simulink model "paramAB_model"  (Simulink 9.3)
settings: Solver=ode23s  StartTime=0.0  StopTime=8  RelTol=1e-3  EnableMultiTasking=on
values from neighbouring files (symbols this model uses):
  model = init_param.model    [paramAB_MPC.m]
undefined symbols (not defined in the file or in its folder): control, simulate
settings Model: Creator=johwa  LastModifiedBy=Jonte  ExtModeAutoUpdateStatusClock=off
settings SolverCC: ConsecutiveZCsStepRelTol=eps
settings DataIOCC: SaveFinalState=on  SignalLoggingName=sigsOut
settings OptimizationCC: ExpressionDepthLimit=2147483647  InitFltsAndDblsToZero=on
settings DebuggingCC: SaveWithParameterizedLinksMsg=none  SignalResolutionControl=TryResolveAllWithWarning  MultiTaskDSMMsg=warning  MultiTaskCondExecSysMsg=none  StateNameClashWarn=warning
settings HardwareCC: TargetUnknown=on
settings GRTTargetCC: TargetFcnLib=ansi_tfl_tmw.mat  GeneratePreprocessorConditionals=Disable all

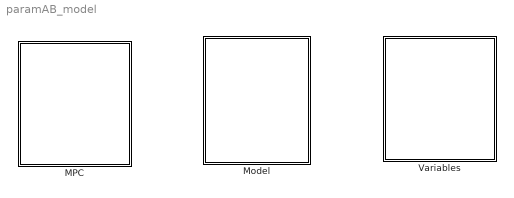
== system paramAB_model ==
  MPC : Subsystem
  Model : Subsystem
  Variables : Subsystem

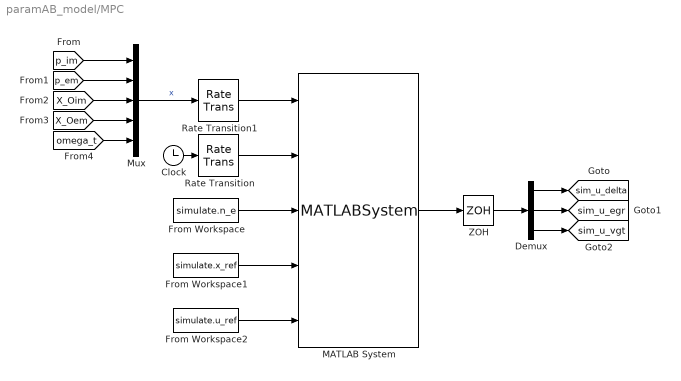
== system paramAB_model/MPC ==
  Clock : Clock
  Demux : Demux  Outputs=3
  From Workspace : FromWorkspace  VariableName=simulate.n_e  SampleTime=simulate.T_s  Interpolate=off  OutputAfterFinalValue=Holding final value
  From Workspace1 : FromWorkspace  VariableName=simulate.x_ref  SampleTime=simulate.T_s  Interpolate=off  OutputAfterFinalValue=Holding final value
  From Workspace2 : FromWorkspace  VariableName=simulate.u_ref  SampleTime=simulate.T_s  Interpolate=off  OutputAfterFinalValue=Holding final value
  MATLAB System : MATLABSystem  System=paramAB_MPC  SimulateUsing=Interpreted execution
      mask Type: paramAB_MPC
      mask Display:
      | disp('paramAB_MPC');
      | port_label('input',1,'x');
      | port_label('input',2,'t');
      | port_label('input',3,'n_e');
      | port_label('input',4,'x_ref');
      | port_label('input',5,'u_ref');
      | port_label('output',1,'u');
  Mux : Mux  Inputs=5
  Rate Transition : RateTransition  OutPortSampleTime=simulate.T_s
  Rate Transition1 : RateTransition  OutPortSampleTime=simulate.T_s
  ZOH : ZeroOrderHold  SampleTime=simulate.T_s
  tag scope: sim_u_delta=global, sim_u_egr=global, sim_u_vgt=global
  wires:
  [omega_t] -> Mux/5
  [X_Oim] -> Mux/3
  [p_im] -> Mux/1
  [p_em] -> Mux/2
  [X_Oem] -> Mux/4
  Clock/1 -> Rate Transition/1
  Rate Transition/1 -> MATLAB System/2
  Demux/2 -> [sim_u_egr]
  Demux/1 -> [sim_u_delta]
  Demux/3 -> [sim_u_vgt]
  MATLAB System/1 -> ZOH/1
  ZOH/1 -> Demux/1
  Mux/1 -> Rate Transition1/1  "x"
  Rate Transition1/1 -> MATLAB System/1
  From Workspace1/1 -> MATLAB System/4
  From Workspace2/1 -> MATLAB System/5
  From Workspace/1 -> MATLAB System/3

== system paramAB_model/Model ==
  Engine : Subsystem  mask{gamma_e=model.gamma_e, gamma_a=model.gamma_a, p_amb=model.p_amb, c_ve=model.c_ve, c_va=model.c_va, c_pe=model.c_pe, c_pa=model.c_pa, T_im=model.T_im, T_amb=model.T_amb, R_e=model.R_e, R_a=model.R_a, X_Oc=model.X_Oc}
      mask help:
      | A model for a Diesel engine with EGT and VGT.
      |
      | The model is develped and parameterized for a Scania heavy duty truck engine and documented in the paper:
      |
      | Johan Wahlstrom and Lars Eriksson.
      | Modeling diesel engines with a variable-geometry turbocharger and exhaust gas recirculation by optimization of model parameters for capturing non-linear system dynamics.
      | Proceedings of the Institution of Mechanical Engineers, Part D, Journal of Automobile Engineering, Volume 225, Issue 7, July 2011.
      | http://dx.doi.org/10.1177/0954407011398177
      mask Help: To see the details of the model right click on the model select "Look Under Mask".
  From Workspace3 : FromWorkspace  VariableName=simulate.n_e  SampleTime=0  Interpolate=off  OutputAfterFinalValue=Holding final value
  wires:
  From Workspace3/1 -> Engine/4(n_e)
  [sim_u_delta] -> Engine/3(u_delta)
  [sim_u_egr] -> Engine/2(u_egr)
  [sim_u_vgt] -> Engine/1(u_vgt)

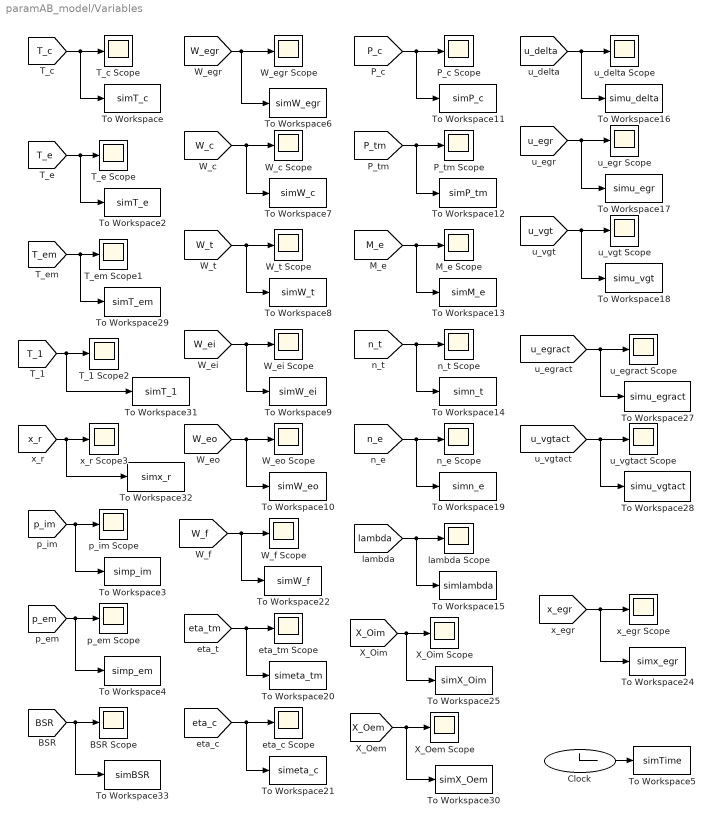
== system paramAB_model/Variables ==
  BSR Scope : Scope
  Clock : Clock
  M_e Scope : Scope
  P_c Scope : Scope
  P_tm Scope : Scope
  T_1 Scope2 : Scope
  T_c Scope : Scope
  T_e Scope : Scope
  T_em Scope1 : Scope
  To Workspace : ToWorkspace  VariableName=simT_c  SampleTime=-1
  To Workspace10 : ToWorkspace  VariableName=simW_eo  SampleTime=-1
  To Workspace11 : ToWorkspace  VariableName=simP_c  SampleTime=-1
  To Workspace12 : ToWorkspace  VariableName=simP_tm  SampleTime=-1
  To Workspace13 : ToWorkspace  VariableName=simM_e  SampleTime=-1
  To Workspace14 : ToWorkspace  VariableName=simn_t  SampleTime=-1
  To Workspace15 : ToWorkspace  VariableName=simlambda  SampleTime=-1
  To Workspace16 : ToWorkspace  VariableName=simu_delta  SampleTime=-1
  To Workspace17 : ToWorkspace  VariableName=simu_egr  SampleTime=-1
  To Workspace18 : ToWorkspace  VariableName=simu_vgt  SampleTime=-1
  To Workspace19 : ToWorkspace  VariableName=simn_e  SampleTime=-1
  To Workspace2 : ToWorkspace  VariableName=simT_e  SampleTime=-1
  To Workspace20 : ToWorkspace  VariableName=simeta_tm  SampleTime=-1
  To Workspace21 : ToWorkspace  VariableName=simeta_c  SampleTime=-1
  To Workspace22 : ToWorkspace  VariableName=simW_f  SampleTime=-1
  To Workspace24 : ToWorkspace  VariableName=simx_egr  SampleTime=-1
  To Workspace25 : ToWorkspace  VariableName=simX_Oim  SampleTime=-1
  To Workspace27 : ToWorkspace  VariableName=simu_egract  SampleTime=-1
  To Workspace28 : ToWorkspace  VariableName=simu_vgtact  SampleTime=-1
  To Workspace29 : ToWorkspace  VariableName=simT_em  SampleTime=-1
  To Workspace3 : ToWorkspace  VariableName=simp_im  SampleTime=-1
  To Workspace30 : ToWorkspace  VariableName=simX_Oem  SampleTime=-1
  To Workspace31 : ToWorkspace  VariableName=simT_1  SampleTime=-1
  To Workspace32 : ToWorkspace  VariableName=simx_r  SampleTime=-1
  To Workspace33 : ToWorkspace  VariableName=simBSR  SampleTime=-1
  To Workspace4 : ToWorkspace  VariableName=simp_em  SampleTime=-1
  To Workspace5 : ToWorkspace  VariableName=simTime  SampleTime=-1
  To Workspace6 : ToWorkspace  VariableName=simW_egr  SampleTime=-1
  To Workspace7 : ToWorkspace  VariableName=simW_c  SampleTime=-1
  To Workspace8 : ToWorkspace  VariableName=simW_t  SampleTime=-1
  To Workspace9 : ToWorkspace  VariableName=simW_ei  SampleTime=-1
  W_c Scope : Scope
  W_egr Scope : Scope
  W_ei Scope : Scope
  W_eo Scope : Scope
  W_f Scope : Scope
  W_t Scope : Scope
  X_Oem Scope : Scope
  X_Oim Scope : Scope
  eta_c Scope : Scope
  eta_tm Scope : Scope
  lambda Scope : Scope
  n_e Scope : Scope
  n_t Scope : Scope
  p_em Scope : Scope
  p_im Scope : Scope
  u_delta Scope : Scope
  u_egr Scope : Scope
  u_egract Scope : Scope
  u_vgt Scope : Scope
  u_vgtact Scope : Scope
  x_egr Scope : Scope
  x_r Scope3 : Scope
  wires:
  [u_vgtact] -> To Workspace28/1, u_vgtact Scope/1
  [u_egract] -> u_egract Scope/1, To Workspace27/1
  [x_egr] -> x_egr Scope/1, To Workspace24/1
  [W_f] -> W_f Scope/1, To Workspace22/1
  [eta_c] -> To Workspace21/1, eta_c Scope/1
  [eta_tm] -> eta_tm Scope/1, To Workspace20/1
  [n_e] -> n_e Scope/1, To Workspace19/1
  [u_vgt] -> u_vgt Scope/1, To Workspace18/1
  [u_egr] -> To Workspace17/1, u_egr Scope/1
  [u_delta] -> u_delta Scope/1, To Workspace16/1
  Clock/1 -> To Workspace5/1
  [lambda] -> To Workspace15/1, lambda Scope/1
  [M_e] -> To Workspace13/1, M_e Scope/1
  [W_eo] -> To Workspace10/1, W_eo Scope/1
  [P_tm] -> To Workspace12/1, P_tm Scope/1
  [P_c] -> To Workspace11/1, P_c Scope/1
  [W_ei] -> To Workspace9/1, W_ei Scope/1
  [W_t] -> To Workspace8/1, W_t Scope/1
  [W_c] -> To Workspace7/1, W_c Scope/1
  [W_egr] -> To Workspace6/1, W_egr Scope/1
  [n_t] -> To Workspace14/1, n_t Scope/1
  [p_em] -> To Workspace4/1, p_em Scope/1
  [p_im] -> To Workspace3/1, p_im Scope/1
  [T_e] -> To Workspace2/1, T_e Scope/1
  [T_c] -> To Workspace/1, T_c Scope/1
  [T_em] -> T_em Scope1/1, To Workspace29/1
  [X_Oem] -> X_Oem Scope/1, To Workspace30/1
  [X_Oim] -> X_Oim Scope/1, To Workspace25/1
  [T_1] -> T_1 Scope2/1, To Workspace31/1
  [x_r] -> x_r Scope3/1, To Workspace32/1
  [BSR] -> BSR Scope/1, To Workspace33/1

== system paramAB_model/Model/Engine ==
  u_vgt : Inport
  u_egr : Inport  Port=2
  u_delta : Inport  Port=3
  n_e : Inport  Port=4
  Cylinder : Subsystem  mask{n_cyl=model.n_cyl, AFs=model.AFs, q_HV=model.q_HV, V_d=model.V_d, r_c=model.r_c}
  EGR-system : Subsystem  mask{PI_egropt=model.PI_egropt, c_egr=model.c_egr, uInit_egr=simulate.u_egr_Init, A_egrmax=model.A_egrmax}
  Exhaust Manifold : Subsystem  mask{p_em_Init=simulate.p_em_Init, V_em=model.V_em}
  Inlet Manifold temp : Constant  Value=T_im
  Intake Manifold : Subsystem  mask{p_im_Init=simulate.p_im_Init, V_im=model.V_im}
  Turbo : Subsystem
  tag scope: T_c=global
  wires:
  Exhaust Manifold/2(X_Oem) -> Intake Manifold/5(X_Oem)
  Cylinder/4(X_Oe) -> Exhaust Manifold/5(X_Oe)
  Intake Manifold/2(X_Oim) -> Cylinder/3(X_Oim)
  u_delta/1 -> Cylinder/5(u_delta)
  n_e/1 -> Cylinder/4(n_e)
  Turbo/2(T_c) -> [T_c]
  u_vgt/1 -> Turbo/4(u_vgt)
  u_egr/1 -> EGR-system/4(u_egr)
  Cylinder/3(T_em) -> EGR-system/2(T_em), Turbo/3(T_em), Exhaust Manifold/4(T_em)
  Cylinder/1(W_ei) -> Intake Manifold/3(W_ei)
  Inlet Manifold temp/1 -> Intake Manifold/4(T_im), Cylinder/6(T_im)
  Turbo/1(W_c) -> Intake Manifold/1(W_c)
  EGR-system/1(W_egr) -> Intake Manifold/2(W_egr), Exhaust Manifold/3(W_egr)
  Turbo/3(W_t) -> Exhaust Manifold/2(W_t)
  Cylinder/2(W_eo) -> Exhaust Manifold/1(W_eo)
  Exhaust Manifold/1(p_em) -> EGR-system/3(p_em), Turbo/2(p_em), Cylinder/2(p_em)
  Intake Manifold/1(p_im) -> EGR-system/1(p_im), Turbo/1(p_im), Cylinder/1(p_im)

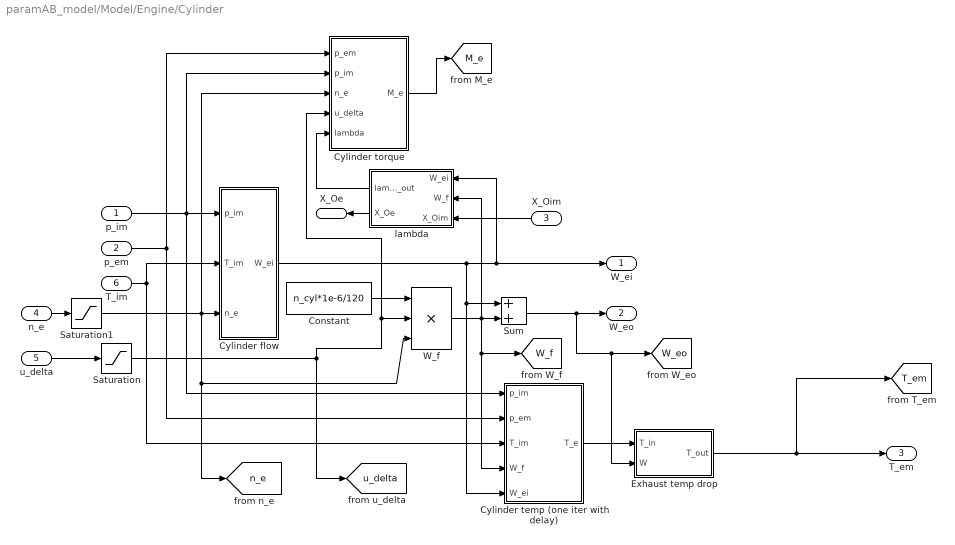
== system paramAB_model/Model/Engine/Cylinder ==
  p_im : Inport
  p_em : Inport  Port=2
  X_Oim : Inport  Port=3
  n_e : Inport  Port=4
  u_delta : Inport  Port=5
  T_im : Inport  Port=6
  Constant : Constant  Value=n_cyl*1e-6/120
  Cylinder flow : Subsystem  mask{c_volVec=model.c_volVec}
  Cylinder temp (one iter with delay) : Subsystem  mask{x_cv=model.x_cv, eta_sc=model.eta_sc, x_r_Init=simulate.x_r_Init, T_1_Init=simulate.T_1_Init}
  Cylinder torque : Subsystem  mask{c_fricVec=model.c_fricVec, eta_igch=model.eta_igch, gamma_c=model.gamma_c}
  Exhaust temp drop : Subsystem  mask{h_tot=model.h_tot, n_pipe=model.n_pipe, l_pipe=model.l_pipe, d_pipe=model.d_pipe, T_w=model.T_w}
  Saturation : Saturate  UpperLimit=250  LowerLimit=1
  Saturation1 : Saturate  UpperLimit=2000  LowerLimit=500
  Sum : Sum  SaturateOnIntegerOverflow=on
  W_f : Product  Inputs=3  SaturateOnIntegerOverflow=on  OutDataTypeStr=Inherit: Same as first input
  lambda : Subsystem
  W_ei : Outport
  W_eo : Outport  Port=2
  T_em : Outport  Port=3
  X_Oe : Outport  Port=4
  tag scope: M_e=global, T_em=global, W_eo=global, W_f=global, n_e=global, u_delta=global
  wires:
  Saturation/1 -> W_f/2, Cylinder torque/4(u_delta), [u_delta]
  lambda/2(X_Oe) -> X_Oe/1
  n_e/1 -> Saturation1/1
  X_Oim/1 -> lambda/3(X_Oim)
  lambda/1(lambda_out) -> Cylinder torque/5(lambda)
  Cylinder temp (one iter with delay)/1(T_e) -> Exhaust temp drop/1(T_in)
  Cylinder torque/1(M_e) -> [M_e]
  u_delta/1 -> Saturation/1
  Constant/1 -> W_f/1
  W_f/1 -> lambda/2(W_f), [W_f], Cylinder temp (one iter with delay)/4(W_f), Sum/2
  Sum/1 -> Exhaust temp drop/2(W), [W_eo], W_eo/1
  Cylinder flow/1(W_ei) -> lambda/1(W_ei), W_ei/1, Cylinder temp (one iter with delay)/5(W_ei), Sum/1
  T_im/1 -> Cylinder flow/2(T_im), Cylinder temp (one iter with delay)/3(T_im)
  p_em/1 -> Cylinder torque/1(p_em), Cylinder temp (one iter with delay)/2(p_em)
  p_im/1 -> Cylinder torque/2(p_im), Cylinder temp (one iter with delay)/1(p_im), Cylinder flow/1(p_im)
  Exhaust temp drop/1(T_out) -> [T_em], T_em/1
  Saturation1/1 -> Cylinder flow/3(n_e), [n_e], W_f/3, Cylinder torque/3(n_e)

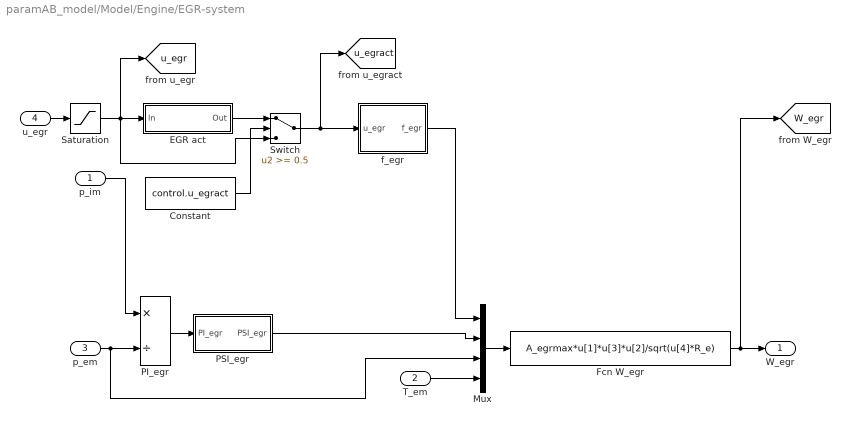
== system paramAB_model/Model/Engine/EGR-system ==
  p_im : Inport
  T_em : Inport  Port=2
  p_em : Inport  Port=3
  u_egr : Inport  Port=4
  Constant : Constant  Value=control.u_egract
  EGR act : Subsystem
  Fcn W_egr : Fcn  Expr=A_egrmax*u[1]*u[3]*u[2]/sqrt(u[4]*R_e)
  Mux : Mux
  PI_egr : Product  Inputs=*/  SaturateOnIntegerOverflow=on  OutDataTypeStr=Inherit: Same as first input
  PSI_egr : Subsystem
  Saturation : Saturate  UpperLimit=100  LowerLimit=0
  Switch : Switch  Threshold=0.5  SaturateOnIntegerOverflow=on
  f_egr : Subsystem
  W_egr : Outport
  tag scope: W_egr=global, u_egr=global, u_egract=global
  wires:
  Constant/1 -> Switch/2
  EGR act/1(Out) -> Switch/1
  Switch/1 -> [u_egract], f_egr/1(u_egr)
  u_egr/1 -> Saturation/1
  Fcn W_egr/1 -> [W_egr], W_egr/1
  T_em/1 -> Mux/4
  PSI_egr/1(PSI_egr) -> Mux/2
  f_egr/1(f_egr) -> Mux/1
  Mux/1 -> Fcn W_egr/1
  PI_egr/1 -> PSI_egr/1(PI_egr)
  p_em/1 -> Mux/3, PI_egr/2
  p_im/1 -> PI_egr/1
  Saturation/1 -> EGR act/1(In), Switch/3, [u_egr]

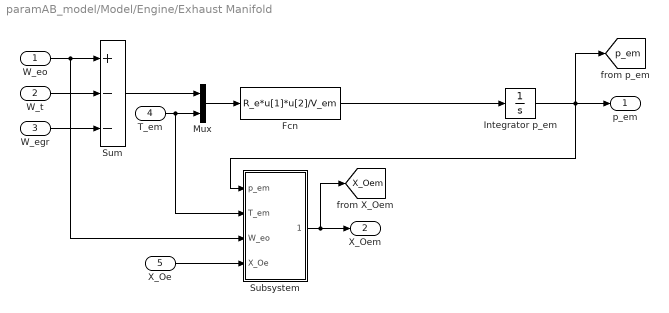
== system paramAB_model/Model/Engine/Exhaust Manifold ==
  W_eo : Inport
  W_t : Inport  Port=2
  W_egr : Inport  Port=3
  T_em : Inport  Port=4
  X_Oe : Inport  Port=5
  Fcn : Fcn  Expr=R_e*u[1]*u[2]/V_em
  Integrator p_em : Integrator  InitialCondition=p_em_Init  LimitOutput=on  UpperSaturationLimit=20*p_amb  LowerSaturationLimit=0.5*p_amb
  Mux : Mux  Inputs=2
  Subsystem : Subsystem
  Sum : Sum  Inputs=+--  SaturateOnIntegerOverflow=on
  p_em : Outport
  X_Oem : Outport  Port=2
  tag scope: X_Oem=global, p_em=global
  wires:
  Subsystem/1(X_Oem) -> [X_Oem], X_Oem/1
  X_Oe/1 -> Subsystem/4(X_Oe)
  Integrator p_em/1 -> Subsystem/1(p_em), [p_em], p_em/1
  W_eo/1 -> Subsystem/3(W_eo), Sum/1
  W_t/1 -> Sum/2
  W_egr/1 -> Sum/3
  Sum/1 -> Mux/1
  T_em/1 -> Subsystem/2(T_em), Mux/2
  Mux/1 -> Fcn/1
  Fcn/1 -> Integrator p_em/1

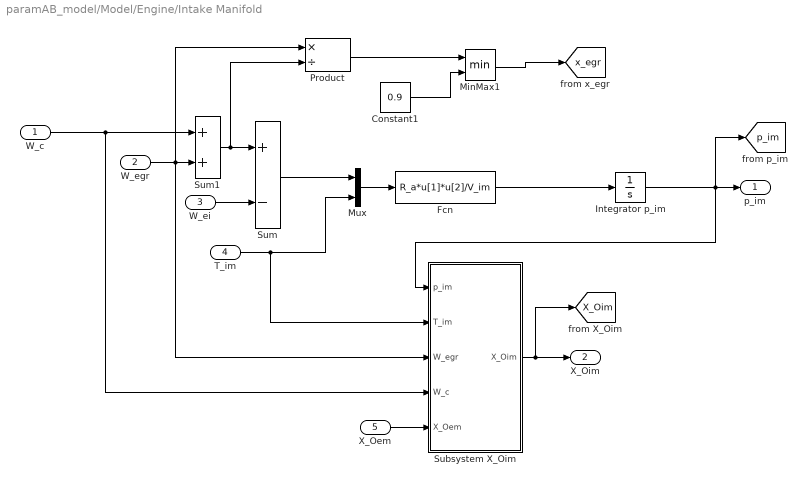
== system paramAB_model/Model/Engine/Intake Manifold ==
  W_c : Inport
  W_egr : Inport  Port=2
  W_ei : Inport  Port=3
  T_im : Inport  Port=4
  X_Oem : Inport  Port=5
  Constant1 : Constant  Value=0.9
  Fcn : Fcn  Expr=R_a*u[1]*u[2]/V_im
  Integrator p_im : Integrator  InitialCondition=p_im_Init  LimitOutput=on  UpperSaturationLimit=10*p_amb  LowerSaturationLimit=0.5*p_amb
  MinMax1 : MinMax  Inputs=2  SaturateOnIntegerOverflow=on  InputSameDT=on
  Mux : Mux  Inputs=2
  Product : Product  Inputs=*/  SaturateOnIntegerOverflow=on  OutDataTypeStr=Inherit: Same as first input
  Subsystem X_Oim : Subsystem
  Sum : Sum  Inputs=+-  SaturateOnIntegerOverflow=on
  Sum1 : Sum  SaturateOnIntegerOverflow=on
  p_im : Outport
  X_Oim : Outport  Port=2
  tag scope: X_Oim=global, p_im=global, x_egr=global
  wires:
  Subsystem X_Oim/1(X_Oim) -> [X_Oim], X_Oim/1
  X_Oem/1 -> Subsystem X_Oim/5(X_Oem)
  Product/1 -> MinMax1/1
  Constant1/1 -> MinMax1/2
  W_egr/1 -> Subsystem X_Oim/3(W_egr), Product/1, Sum1/2
  W_c/1 -> Subsystem X_Oim/4(W_c), Sum1/1
  Sum1/1 -> Product/2, Sum/1
  Fcn/1 -> Integrator p_im/1
  Mux/1 -> Fcn/1
  T_im/1 -> Subsystem X_Oim/2(T_im), Mux/2
  Sum/1 -> Mux/1
  W_ei/1 -> Sum/2
  Integrator p_im/1 -> Subsystem X_Oim/1(p_im), [p_im], p_im/1
  MinMax1/1 -> [x_egr]

== system paramAB_model/Model/Engine/Turbo ==
  p_im : Inport
  p_em : Inport  Port=2
  T_em : Inport  Port=3
  u_vgt : Inport  Port=4
  Compressor : Subsystem  mask{c_pi=model.c_pi, pi_copt=model.pi_copt, w_copt=model.w_copt, eta_cmax=model.eta_cmax, Q_c=model.Q_c, c_wphiVec=model.c_wphiVec, c_wpsiVec=model.c_wpsiVec, c_phi2=model.c_phi2, c_psi2=model.c_psi2, R_c=model.R_c}
  Turbine : Subsystem  mask{c_vgt2=model.c_vgt2, c_vgt1=model.c_vgt1, c_f2=model.c_f2, c_f1=model.c_f1, K_t=model.K_t, uInit_vgt=simulate.u_vgt_Init, tau_vgt=model.tau_vgt, c_mlin=model.c_mlin, w_tlin=model.w_tlin, c_mVec=model.c_mVec, BSR_opt=model.BSR_opt, eta_tmmax=model.eta_tmmax, R_t=model.R_t, A_vgtmax=model.A_vgtmax}
  Turbo inertia : Subsystem  mask{omega_t_Init=simulate.omega_t_Init, J_t=model.J_t}
  amb pres : Constant  Value=p_amb
  amb temp : Constant  Value=T_amb
  W_c : Outport
  T_c : Outport  Port=2
  W_t : Outport  Port=3
  wires:
  u_vgt/1 -> Turbine/5(u_vgt)
  T_em/1 -> Turbine/1(T_em)
  p_em/1 -> Turbine/2(p_em)
  Turbine/1(W_t) -> W_t/1
  Compressor/2(T_c) -> T_c/1
  Compressor/1(W_c) -> W_c/1
  Compressor/3(P_c) -> Turbo inertia/2(P_c)
  Turbine/2(P_t*eta_m) -> Turbo inertia/1(P_t*eta_m)
  Turbo inertia/1(omega_t) -> Turbine/4(omega_t), Compressor/4(omega_t)
  p_im/1 -> Compressor/3(p_c)
  amb pres/1 -> Turbine/3(p_es), Compressor/2(p_bc)
  amb temp/1 -> Compressor/1(T_bc)

== system paramAB_model/Model/Engine/Cylinder/Cylinder flow ==
  p_im : Inport
  T_im : Inport  Port=2
  n_e : Inport  Port=3
  Constant : Constant  Value=V_d/(R_a*60*2)
  Mux : Mux  Inputs=2
  Product W_ei : Product  Inputs=***/*  SaturateOnIntegerOverflow=on  OutDataTypeStr=Inherit: Same as first input
  n_vol : Fcn  Expr=c_volVec(1)*sqrt(u[1])+c_volVec(2)*sqrt(u[2])+c_volVec(3)
  W_ei : Outport
  tag scope: W_ei=global
  wires:
  Mux/1 -> n_vol/1
  Product W_ei/1 -> [W_ei], W_ei/1
  Constant/1 -> Product W_ei/5
  T_im/1 -> Product W_ei/4
  n_e/1 -> Mux/2, Product W_ei/3
  n_vol/1 -> Product W_ei/1
  p_im/1 -> Mux/1, Product W_ei/2

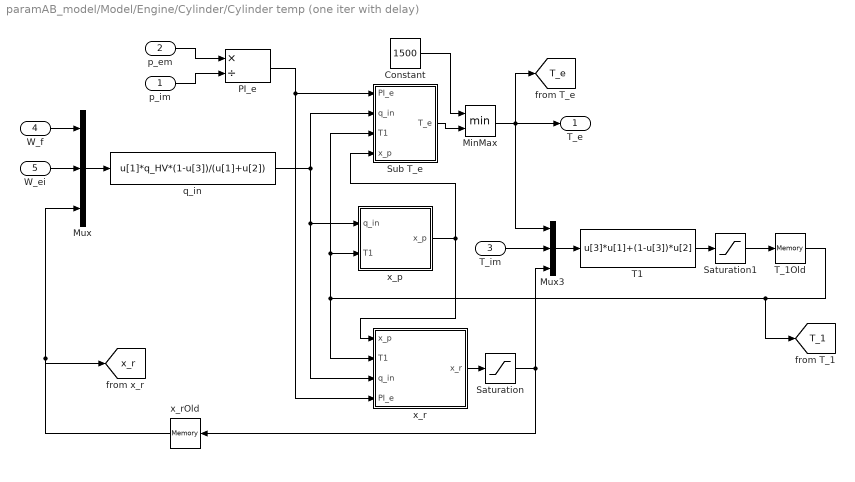
== system paramAB_model/Model/Engine/Cylinder/Cylinder temp (one iter with delay) ==
  p_im : Inport
  p_em : Inport  Port=2
  T_im : Inport  Port=3
  W_f : Inport  Port=4
  W_ei : Inport  Port=5
  Constant : Constant  Value=1500
  MinMax : MinMax  Inputs=2  SaturateOnIntegerOverflow=on  InputSameDT=on
  Mux : Mux  Inputs=3
  Mux3 : Mux  Inputs=3
  PI_e : Product  Inputs=*/  SaturateOnIntegerOverflow=on  OutDataTypeStr=Inherit: Same as first input
  Saturation : Saturate  UpperLimit=1  LowerLimit=0
  Saturation1 : Saturate  UpperLimit=inf  LowerLimit=273
  Sub T_e : Subsystem
  T1 : Fcn  Expr=u[3]*u[1]+(1-u[3])*u[2]
  T_1Old : Memory  InitialCondition=T_1_Init  InheritSampleTime=on
  q_in : Fcn  Expr=u[1]*q_HV*(1-u[3])/(u[1]+u[2])
  x_p : Subsystem
  x_r : Subsystem
  x_rOld : Memory  InitialCondition=x_r_Init  InheritSampleTime=on
  T_e : Outport
  tag scope: T_1=global, T_e=global, x_r=global
  wires:
  Saturation1/1 -> T_1Old/1
  Saturation/1 -> x_rOld/1, Mux3/3
  Constant/1 -> MinMax/1
  Sub T_e/1(T_e) -> MinMax/2
  MinMax/1 -> [T_e], Mux3/1, T_e/1
  x_rOld/1 -> [x_r], Mux/3
  x_r/1(x_r) -> Saturation/1
  T_1Old/1 -> [T_1], x_r/2(T1), x_p/2(T1), Sub T_e/3(T1)
  T1/1 -> Saturation1/1
  T_im/1 -> Mux3/2
  Mux3/1 -> T1/1
  x_p/1(x_p) -> x_r/1(x_p), Sub T_e/4(x_p)
  PI_e/1 -> x_r/4(PI_e), Sub T_e/1(PI_e)
  q_in/1 -> Sub T_e/2(q_in), x_p/1(q_in), x_r/3(q_in)
  W_ei/1 -> Mux/2
  W_f/1 -> Mux/1
  Mux/1 -> q_in/1
  p_em/1 -> PI_e/1
  p_im/1 -> PI_e/2

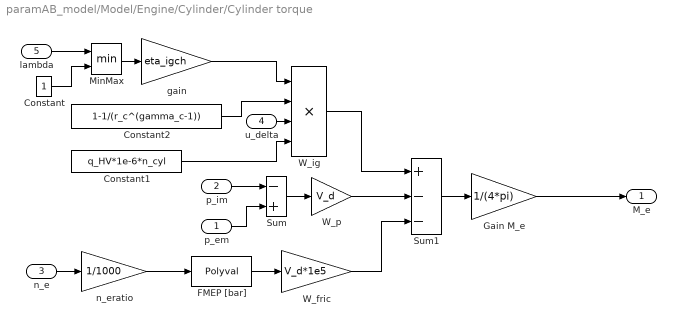
== system paramAB_model/Model/Engine/Cylinder/Cylinder torque ==
  p_em : Inport
  p_im : Inport  Port=2
  n_e : Inport  Port=3
  u_delta : Inport  Port=4
  lambda : Inport  Port=5
  Constant : Constant
  Constant1 : Constant  Value=q_HV*1e-6*n_cyl
  Constant2 : Constant  Value=1-1/(r_c^(gamma_c-1))
  FMEP [bar] : Polyval  Coefs=c_fricVec
  Gain M_e : Gain  Gain=1/(4*pi)  SaturateOnIntegerOverflow=on  OutDataTypeStr=Inherit: Same as input  ParamDataTypeStr=Inherit: Same as input
  MinMax : MinMax  Inputs=2  SaturateOnIntegerOverflow=on  InputSameDT=on
  Sum : Sum  Inputs=-+  SaturateOnIntegerOverflow=on
  Sum1 : Sum  Inputs=+--  SaturateOnIntegerOverflow=on
  W_fric : Gain  Gain=V_d*1e5  SaturateOnIntegerOverflow=on  OutDataTypeStr=Inherit: Same as input  ParamDataTypeStr=Inherit: Same as input
  W_ig : Product  Inputs=4  SaturateOnIntegerOverflow=on  OutDataTypeStr=Inherit: Same as first input
  W_p : Gain  Gain=V_d  SaturateOnIntegerOverflow=on  OutDataTypeStr=Inherit: Same as input  ParamDataTypeStr=Inherit: Same as input
  gain : Gain  Gain=eta_igch  SaturateOnIntegerOverflow=on  OutDataTypeStr=Inherit: Same as input  ParamDataTypeStr=Inherit: Same as input
  n_eratio : Gain  Gain=1/1000  SaturateOnIntegerOverflow=on  OutDataTypeStr=Inherit: Same as input  ParamDataTypeStr=Inherit: Same as input
  M_e : Outport
  wires:
  Gain M_e/1 -> M_e/1
  Constant1/1 -> W_ig/4
  u_delta/1 -> W_ig/3
  Constant2/1 -> W_ig/2
  Sum1/1 -> Gain M_e/1
  W_fric/1 -> Sum1/3
  W_p/1 -> Sum1/2
  W_ig/1 -> Sum1/1
  FMEP [bar]/1 -> W_fric/1
  n_eratio/1 -> FMEP [bar]/1
  n_e/1 -> n_eratio/1
  gain/1 -> W_ig/1
  MinMax/1 -> gain/1
  Constant/1 -> MinMax/2
  lambda/1 -> MinMax/1
  Sum/1 -> W_p/1
  p_em/1 -> Sum/2
  p_im/1 -> Sum/1

== system paramAB_model/Model/Engine/Cylinder/Exhaust temp drop ==
  T_in : Inport
  W : Inport  Port=2
  Fcn T_out : Fcn  Expr=T_w+(u[1]-T_w)*exp(-1*h_tot*pi*d_pipe*l_pipe*n_pipe/(u[2]*c_pe))
  Mux : Mux  Inputs=2
  T_out : Outport
  wires:
  Fcn T_out/1 -> T_out/1
  Mux/1 -> Fcn T_out/1
  W/1 -> Mux/2
  T_in/1 -> Mux/1

== system paramAB_model/Model/Engine/Cylinder/lambda ==
  W_ei : Inport
  W_f : Inport  Port=2
  X_Oim : Inport  Port=3
  Constant1 : Constant  Value=AFs*X_Oc
  Constant2 : Constant  Value=0
  Fcn : Fcn  Expr=(u[1]*u[3]-u[2]*AFs*X_Oc)/(u[1]+u[2])
  MinMax : MinMax  Function=max  Inputs=2  SaturateOnIntegerOverflow=on  InputSameDT=on
  Mux : Mux  Inputs=3
  lambda : Product  Inputs=/*/*  SaturateOnIntegerOverflow=on  OutDataTypeStr=Inherit: Same as first input
  lambda_out : Outport
  X_Oe : Outport  Port=2
  tag scope: lambda=global
  wires:
  Constant2/1 -> MinMax/2
  Fcn/1 -> MinMax/1
  MinMax/1 -> X_Oe/1
  Mux/1 -> Fcn/1
  X_Oim/1 -> Mux/3, lambda/4
  W_f/1 -> Mux/2, lambda/3
  W_ei/1 -> Mux/1, lambda/2
  lambda/1 -> lambda_out/1, [lambda]
  Constant1/1 -> lambda/1

== system paramAB_model/Model/Engine/EGR-system/EGR act ==
  In : Inport
  Actuator1 : Subsystem  mask{tau=model.tau_egr1, uInit=simulate.utilde_egr1_Init}
  Actuator2 : Subsystem  mask{tau=model.tau_egr2, uInit=simulate.utilde_egr2_Init}
  Gain : Gain  Gain=model.K_egr
  Gain1 : Gain  Gain=model.K_egr-1
  Subtract : Sum  Inputs=+-
  Transport Delay : TransportDelay  DelayTime=model.tau_degr  InitialOutput=model.uInit_egr
  Out : Outport
  wires:
  Gain1/1 -> Subtract/2
  Gain/1 -> Subtract/1
  Actuator2/1(Out) -> Gain1/1
  Actuator1/1(Out) -> Gain/1
  Transport Delay/1 -> Actuator2/1(In), Actuator1/1(In)
  Subtract/1 -> Out/1
  In/1 -> Transport Delay/1

== system paramAB_model/Model/Engine/EGR-system/PSI_egr ==
  PI_egr : Inport
  PSI_egr function : Fcn  Expr=1-((1-u)/(1-PI_egropt)-1)^2
  Saturation : Saturate  UpperLimit=1  LowerLimit=PI_egropt
  PSI_egr : Outport
  wires:
  PSI_egr function/1 -> PSI_egr/1
  PI_egr/1 -> Saturation/1
  Saturation/1 -> PSI_egr function/1

== system paramAB_model/Model/Engine/EGR-system/f_egr ==
  u_egr : Inport
  Constant : Constant  Value=0
  Constant1 : Constant  Value=-c_egr(2)/2/c_egr(1)
  MinMax : MinMax  Function=max  Inputs=2  SaturateOnIntegerOverflow=on  InputSameDT=on
  MinMax1 : MinMax  Inputs=2  SaturateOnIntegerOverflow=on  InputSameDT=on
  Polynomial : Polyval  Coefs=c_egr
  f_egr : Outport
  wires:
  Constant1/1 -> MinMax1/2
  MinMax1/1 -> Polynomial/1
  u_egr/1 -> MinMax1/1
  MinMax/1 -> f_egr/1
  Constant/1 -> MinMax/2
  Polynomial/1 -> MinMax/1

== system paramAB_model/Model/Engine/Exhaust Manifold/Subsystem ==
  p_em : Inport
  T_em : Inport  Port=2
  W_eo : Inport  Port=3
  X_Oe : Inport  Port=4
  Fcn1 : Fcn  Expr=R_e*u[2]/u[1]/V_em*u[3]*(u[4]-u[5])
  Integrator X_Oem : Integrator  InitialCondition=simulate.X_Oem_Init  LimitOutput=on  UpperSaturationLimit=1  LowerSaturationLimit=0
  Mux1 : Mux  Inputs=5
  X_Oem : Outport
  wires:
  T_em/1 -> Mux1/2
  X_Oe/1 -> Mux1/4
  Integrator X_Oem/1 -> Mux1/5, X_Oem/1
  W_eo/1 -> Mux1/3
  p_em/1 -> Mux1/1
  Fcn1/1 -> Integrator X_Oem/1
  Mux1/1 -> Fcn1/1

== system paramAB_model/Model/Engine/Intake Manifold/Subsystem X_Oim ==
  p_im : Inport
  T_im : Inport  Port=2
  W_egr : Inport  Port=3
  W_c : Inport  Port=4
  X_Oem : Inport  Port=5
  Fcn1 : Fcn  Expr=R_a*u[2]/u[1]/V_im*(u[3]*(u[5]-u[6])+u[4]*(X_Oc-u[6]))
  Integrator X_Oim : Integrator  InitialCondition=simulate.X_Oim_Init  LimitOutput=on  UpperSaturationLimit=1  LowerSaturationLimit=0
  Mux1 : Mux  Inputs=6
  X_Oim : Outport
  wires:
  X_Oem/1 -> Mux1/5
  Integrator X_Oim/1 -> Mux1/6, X_Oim/1
  W_c/1 -> Mux1/4
  W_egr/1 -> Mux1/3
  T_im/1 -> Mux1/2
  p_im/1 -> Mux1/1
  Mux1/1 -> Fcn1/1
  Fcn1/1 -> Integrator X_Oim/1

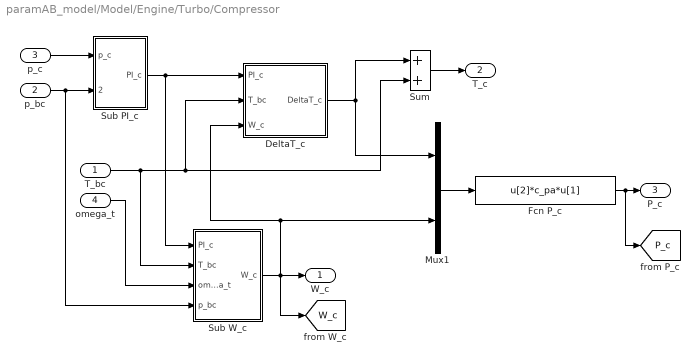
== system paramAB_model/Model/Engine/Turbo/Compressor ==
  T_bc : Inport
  p_bc : Inport  Port=2
  p_c : Inport  Port=3
  omega_t : Inport  Port=4
  DeltaT_c : Subsystem
  Fcn P_c : Fcn  Expr=u[2]*c_pa*u[1]
  Mux1 : Mux  Inputs=2
  Sub PI_c : Subsystem
  Sub W_c : Subsystem
  Sum : Sum  SaturateOnIntegerOverflow=on
  W_c : Outport
  T_c : Outport  Port=2
  P_c : Outport  Port=3
  tag scope: P_c=global, W_c=global
  wires:
  Sum/1 -> T_c/1
  Fcn P_c/1 -> [P_c], P_c/1
  Sub W_c/1(W_c) -> [W_c], DeltaT_c/3(W_c), Mux1/2, W_c/1
  omega_t/1 -> Sub W_c/3(omega_t)
  T_bc/1 -> Sub W_c/2(T_bc), DeltaT_c/2(T_bc), Sum/2
  Mux1/1 -> Fcn P_c/1
  DeltaT_c/1(DeltaT_c) -> Sum/1, Mux1/1
  Sub PI_c/1(PI_c) -> DeltaT_c/1(PI_c), Sub W_c/1(PI_c)
  p_bc/1 -> Sub PI_c/2(p_bc), Sub W_c/4(p_bc)
  p_c/1 -> Sub PI_c/1(p_c)

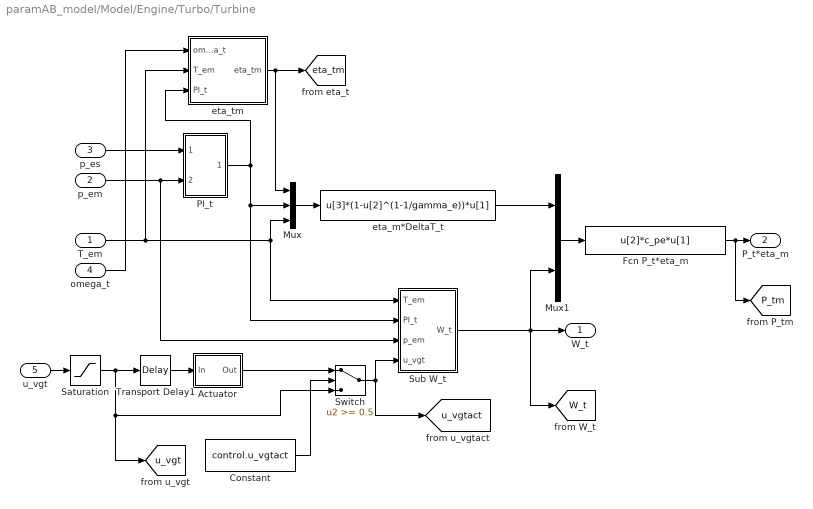
== system paramAB_model/Model/Engine/Turbo/Turbine ==
  T_em : Inport
  p_em : Inport  Port=2
  p_es : Inport  Port=3
  omega_t : Inport  Port=4
  u_vgt : Inport  Port=5
  Actuator : Subsystem  mask{tau=tau_vgt, uInit=simulate.utilde_vgt_Init}
  Constant : Constant  Value=control.u_vgtact
  Fcn P_t*eta_m : Fcn  Expr=u[2]*c_pe*u[1]
  Mux : Mux  Inputs=3
  Mux1 : Mux  Inputs=2
  PI_t : Subsystem
  Saturation : Saturate  UpperLimit=100  LowerLimit=20
  Sub W_t : Subsystem
  Switch : Switch  Threshold=0.5  SaturateOnIntegerOverflow=on
  Transport Delay1 : TransportDelay  DelayTime=model.tau_dvgt  InitialOutput=model.uInit_vgt
  eta_m*DeltaT_t : Fcn  Expr=u[3]*(1-u[2]^(1-1/gamma_e))*u[1]
  eta_tm : Subsystem
  W_t : Outport
  P_t*eta_m : Outport  Port=2
  tag scope: P_tm=global, W_t=global, eta_tm=global, u_vgt=global, u_vgtact=global
  wires:
  Switch/1 -> [u_vgtact], Sub W_t/4(u_vgt)
  Actuator/1(Out) -> Switch/1
  Constant/1 -> Switch/2
  Transport Delay1/1 -> Actuator/1(In)
  u_vgt/1 -> Saturation/1
  eta_tm/1(eta_tm) -> [eta_tm], Mux/1
  Sub W_t/1(W_t) -> [W_t], Mux1/2, W_t/1
  p_es/1 -> PI_t/1(p_es)
  p_em/1 -> Sub W_t/3(p_em), PI_t/2(p_em)
  PI_t/1(PI_t) -> eta_tm/3(PI_t), Sub W_t/2(PI_t), Mux/2
  Mux/1 -> eta_m*DeltaT_t/1
  eta_m*DeltaT_t/1 -> Mux1/1
  Mux1/1 -> Fcn P_t*eta_m/1
  T_em/1 -> eta_tm/2(T_em), Mux/3, Sub W_t/1(T_em)
  omega_t/1 -> eta_tm/1(omega_t)
  Fcn P_t*eta_m/1 -> [P_tm], P_t*eta_m/1
  Saturation/1 -> Switch/3, [u_vgt], Transport Delay1/1

== system paramAB_model/Model/Engine/Turbo/Turbo inertia ==
  P_t*eta_m : Inport
  P_c : Inport  Port=2
  Divide : Product  Inputs=*/
  Gain : Gain  Gain=1/J_t  SaturateOnIntegerOverflow=on  OutDataTypeStr=Inherit: Same as input  ParamDataTypeStr=Inherit: Same as input
  Gain2 : Gain  Gain=30/pi  SaturateOnIntegerOverflow=on  OutDataTypeStr=Inherit: Same as input  ParamDataTypeStr=Inherit: Same as input
  Integrator omega_t : Integrator  InitialCondition=omega_t_Init  LimitOutput=on  UpperSaturationLimit=200000*pi/30  LowerSaturationLimit=100*pi/30
  Sum : Sum  Inputs=+-  SaturateOnIntegerOverflow=on
  omega_t : Outport
  tag scope: n_t=global, omega_t=global
  wires:
  Integrator omega_t/1 -> [omega_t], Gain2/1, Divide/2, omega_t/1
  P_c/1 -> Sum/2
  P_t*eta_m/1 -> Sum/1
  Gain2/1 -> [n_t]
  Gain/1 -> Integrator omega_t/1
  Sum/1 -> Divide/1
  Divide/1 -> Gain/1

== system paramAB_model/Model/Engine/Cylinder/Cylinder temp (one iter with delay)/Sub T_e ==
  PI_e : Inport
  q_in : Inport  Port=2
  T1 : Inport  Port=3
  x_p : Inport  Port=4
  Fcn T_e : Fcn  Expr=eta_sc*u[1]^(1-1/gamma_a)*r_c^(1-gamma_a)*u[4]^(1/gamma_a-1)*(u[2]*((1-x_cv)/c_pa+x_cv/c_va)+u[3]*r_c^(gamma_a-1))
  Mux2 : Mux
  T_e : Outport
  wires:
  Fcn T_e/1 -> T_e/1
  x_p/1 -> Mux2/4
  T1/1 -> Mux2/3
  q_in/1 -> Mux2/2
  PI_e/1 -> Mux2/1
  Mux2/1 -> Fcn T_e/1

== system paramAB_model/Model/Engine/Cylinder/Cylinder temp (one iter with delay)/x_p ==
  q_in : Inport
  T1 : Inport  Port=2
  Fcn x_p : Fcn  Expr=1+u[1]*x_cv/(c_va*u[2]*r_c^(gamma_a-1))
  Mux1 : Mux  Inputs=2
  x_p : Outport
  wires:
  Fcn x_p/1 -> x_p/1
  T1/1 -> Mux1/2
  q_in/1 -> Mux1/1
  Mux1/1 -> Fcn x_p/1

== system paramAB_model/Model/Engine/Cylinder/Cylinder temp (one iter with delay)/x_r ==
  x_p : Inport
  T1 : Inport  Port=2
  q_in : Inport  Port=3
  PI_e : Inport  Port=4
  Fcn x_r : Fcn  Expr=u[3]^(1/gamma_a)*u[1]^(-1/gamma_a)/(r_c*u[2])
  Mux4 : Mux  Inputs=2
  Mux5 : Mux  Inputs=3
  x_v : Fcn  Expr=1+u[2]*(1-x_cv)/(c_pa*(u[2]*x_cv/c_va+u[1]*r_c^(gamma_a-1)))
  x_r : Outport
  wires:
  PI_e/1 -> Mux5/3
  q_in/1 -> Mux4/2
  T1/1 -> Mux4/1
  x_p/1 -> Mux5/1
  x_v/1 -> Mux5/2
  Fcn x_r/1 -> x_r/1
  Mux5/1 -> Fcn x_r/1
  Mux4/1 -> x_v/1

== system paramAB_model/Model/Engine/EGR-system/EGR act/Actuator1 ==
  In : Inport
  Gain : Gain  Gain=1/tau  SaturateOnIntegerOverflow=on  OutDataTypeStr=Inherit: Same as input  ParamDataTypeStr=Inherit: Same as input
  Goto : Goto  Commented=on  GotoTag=u_egract1  TagVisibility=global
  Integrator : Integrator  InitialCondition=uInit
  Sum : Sum  Inputs=|+-  SaturateOnIntegerOverflow=on
  Out : Outport
  wires:
  Gain/1 -> Integrator/1
  Sum/1 -> Gain/1
  Integrator/1 -> Sum/2, Out/1
  In/1 -> Sum/1

== system paramAB_model/Model/Engine/EGR-system/EGR act/Actuator2 ==
  In : Inport
  Gain : Gain  Gain=1/tau  SaturateOnIntegerOverflow=on  OutDataTypeStr=Inherit: Same as input  ParamDataTypeStr=Inherit: Same as input
  Goto : Goto  Commented=on  GotoTag=u_egract2  TagVisibility=global
  Integrator : Integrator  InitialCondition=uInit
  Sum : Sum  Inputs=|+-  SaturateOnIntegerOverflow=on
  Out : Outport
  wires:
  Gain/1 -> Integrator/1
  Sum/1 -> Gain/1
  Integrator/1 -> Out/1, Sum/2
  In/1 -> Sum/1

== system paramAB_model/Model/Engine/Turbo/Compressor/DeltaT_c ==
  PI_c : Inport
  T_bc : Inport  Port=2
  W_c : Inport  Port=3
  Fcn DeltaT_c : Fcn  Expr=u[3]*(u[2]^(1-1/gamma_a)-1)/u[1]
  Mux : Mux  Inputs=3
  eta_c : Subsystem
  DeltaT_c : Outport
  tag scope: eta_c=global
  wires:
  Fcn DeltaT_c/1 -> DeltaT_c/1
  T_bc/1 -> Mux/3
  PI_c/1 -> Mux/2, eta_c/2(PI_c)
  W_c/1 -> eta_c/1(W_c)
  eta_c/1(eta_c) -> [eta_c], Mux/1
  Mux/1 -> Fcn DeltaT_c/1

== system paramAB_model/Model/Engine/Turbo/Compressor/Sub PI_c ==
  p_c : Inport
  p_bc : Inport  Port=2
  Constant1 : Constant
  Div PI_c : Product  Inputs=*/  SaturateOnIntegerOverflow=on  OutDataTypeStr=Inherit: Same as first input
  MinMax1 : MinMax  Function=max  Inputs=2  SaturateOnIntegerOverflow=on  InputSameDT=on
  PI_c : Outport
  wires:
  MinMax1/1 -> PI_c/1
  p_c/1 -> Div PI_c/1
  p_bc/1 -> Div PI_c/2
  Constant1/1 -> MinMax1/2
  Div PI_c/1 -> MinMax1/1

== system paramAB_model/Model/Engine/Turbo/Compressor/Sub W_c ==
  PI_c : Inport
  T_bc : Inport  Port=2
  omega_t : Inport  Port=3
  p_bc : Inport  Port=4
  Fcn W_c : Fcn  Expr=u[3]*pi*R_c^3*u[1]*u[4]/(R_a*u[2])
  Mux3 : Mux
  PHI_c : Subsystem
  Saturation : Saturate  UpperLimit=inf  LowerLimit=1e-4
  W_c : Outport
  wires:
  Saturation/1 -> W_c/1
  Fcn W_c/1 -> Saturation/1
  PI_c/1 -> PHI_c/1(PI_c)
  p_bc/1 -> Mux3/3
  T_bc/1 -> Mux3/2, PHI_c/2(T_bc)
  omega_t/1 -> Mux3/1, PHI_c/3(omega_t)
  PHI_c/1(PHI_c) -> Mux3/4
  Mux3/1 -> Fcn W_c/1

== system paramAB_model/Model/Engine/Turbo/Turbine/Actuator ==
  In : Inport
  Gain : Gain  Gain=1/tau  SaturateOnIntegerOverflow=on  OutDataTypeStr=Inherit: Same as input  ParamDataTypeStr=Inherit: Same as input
  Integrator : Integrator  InitialCondition=uInit
  Sum : Sum  Inputs=|+-  SaturateOnIntegerOverflow=on
  Out : Outport
  wires:
  Gain/1 -> Integrator/1
  Sum/1 -> Gain/1
  Integrator/1 -> Sum/2, Out/1
  In/1 -> Sum/1

== system paramAB_model/Model/Engine/Turbo/Turbine/PI_t ==
  p_es : Inport
  p_em : Inport  Port=2
  Constant : Constant  Value=0.9999
  Div PI_t : Product  Inputs=*/  SaturateOnIntegerOverflow=on  OutDataTypeStr=Inherit: Same as first input
  MinMax : MinMax  Inputs=2  SaturateOnIntegerOverflow=on  InputSameDT=on
  PI_t : Outport
  wires:
  MinMax/1 -> PI_t/1
  p_es/1 -> Div PI_t/1
  p_em/1 -> Div PI_t/2
  Div PI_t/1 -> MinMax/1
  Constant/1 -> MinMax/2

== system paramAB_model/Model/Engine/Turbo/Turbine/Sub W_t ==
  T_em : Inport
  PI_t : Inport  Port=2
  p_em : Inport  Port=3
  u_vgt : Inport  Port=4
  Fcn W_t : Fcn  Expr=A_vgtmax*u[3]*sqrt(1-u[2]^K_t)*u[4]/sqrt(u[1]*R_e)
  Mux3 : Mux
  f_vgt : Subsystem
  W_t : Outport
  wires:
  u_vgt/1 -> f_vgt/1(u_vgt)
  Fcn W_t/1 -> W_t/1
  p_em/1 -> Mux3/3
  PI_t/1 -> Mux3/2
  T_em/1 -> Mux3/1
  f_vgt/1(f_vgt) -> Mux3/4
  Mux3/1 -> Fcn W_t/1

== system paramAB_model/Model/Engine/Turbo/Turbine/eta_tm ==
  omega_t : Inport
  T_em : Inport  Port=2
  PI_t : Inport  Port=3
  BSR : Fcn  Expr=R_t*u[1]/sqrt(2*c_pe*u[2]*(1-u[3]^(1-1/gamma_e)))
  Fcn eta_t : Fcn  Expr=eta_tmmax-u[1]*(u[2]-BSR_opt)^2
  Mux1 : Mux  Inputs=2
  Mux4 : Mux  Inputs=3
  Saturation : Saturate  UpperLimit=2*BSR_opt  LowerLimit=0
  Saturation1 : Saturate  UpperLimit=1  LowerLimit=0.2
  c_m : Subsystem
  eta_tm : Outport
  tag scope: BSR=global
  wires:
  c_m/1(c_m) -> Mux1/1
  Saturation/1 -> [BSR], Mux1/2
  Mux1/1 -> Fcn eta_t/1
  Saturation1/1 -> eta_tm/1
  Fcn eta_t/1 -> Saturation1/1
  PI_t/1 -> Mux4/3
  T_em/1 -> Mux4/2
  omega_t/1 -> c_m/1(omega_t), Mux4/1
  BSR/1 -> Saturation/1
  Mux4/1 -> BSR/1

== system paramAB_model/Model/Engine/Turbo/Compressor/DeltaT_c/eta_c ==
  W_c : Inport
  PI_c : Inport  Port=2
  Constant2 : Constant  Value=0.2
  Fcn eta_c : Fcn  Expr=eta_cmax-u
  Matrix Gain : Gain  Gain=Q_c  Multiplication=Matrix(K*u)  SaturateOnIntegerOverflow=on  OutDataTypeStr=Inherit: Same as input  ParamDataTypeStr=Inherit: Same as input
  MinMax2 : MinMax  Function=max  Inputs=2  SaturateOnIntegerOverflow=on  InputSameDT=on
  Mux6 : Mux  Inputs=2
  Product : Product  Multiplication=Matrix(*)  SaturateOnIntegerOverflow=on  OutDataTypeStr=Inherit: Same as first input
  chi1 : Fcn  Expr=u-w_copt
  chi2 : Fcn  Expr=u-pi_copt
  pi_c : Fcn  Expr=(u-1)^c_pi
  transp : Math  Operator=transpose  SaturateOnIntegerOverflow=on
  eta_c : Outport
  wires:
  W_c/1 -> chi1/1
  MinMax2/1 -> eta_c/1
  PI_c/1 -> pi_c/1
  Constant2/1 -> MinMax2/2
  Fcn eta_c/1 -> MinMax2/1
  Product/1 -> Fcn eta_c/1
  Matrix Gain/1 -> Product/2
  transp/1 -> Product/1
  Mux6/1 -> transp/1, Matrix Gain/1
  chi2/1 -> Mux6/2
  chi1/1 -> Mux6/1
  pi_c/1 -> chi2/1

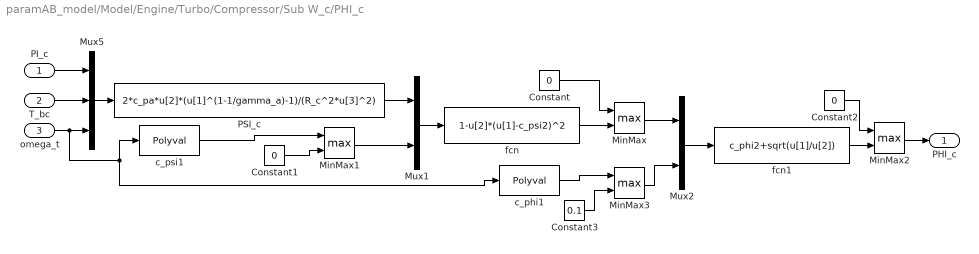
== system paramAB_model/Model/Engine/Turbo/Compressor/Sub W_c/PHI_c ==
  PI_c : Inport
  T_bc : Inport  Port=2
  omega_t : Inport  Port=3
  Constant : Constant  Value=0
  Constant1 : Constant  Value=0
  Constant2 : Constant  Value=0
  Constant3 : Constant  Value=0.1
  MinMax{,1..3} (4 alike) : MinMax  Function=max  Inputs=2  SaturateOnIntegerOverflow=on  InputSameDT=on
  Mux1 : Mux  Inputs=2
  Mux2 : Mux  Inputs=2
  Mux5 : Mux  Inputs=3
  PSI_c : Fcn  Expr=2*c_pa*u[2]*(u[1]^(1-1/gamma_a)-1)/(R_c^2*u[3]^2)
  c_phi1 : Polyval  Coefs=c_wphiVec
  c_psi1 : Polyval  Coefs=c_wpsiVec
  fcn : Fcn  Expr=1-u[2]*(u[1]-c_psi2)^2
  fcn1 : Fcn  Expr=c_phi2+sqrt(u[1]/u[2])
  PHI_c : Outport
  wires:
  Constant3/1 -> MinMax3/2
  MinMax3/1 -> Mux2/2
  c_phi1/1 -> MinMax3/1
  MinMax2/1 -> PHI_c/1
  fcn1/1 -> MinMax2/2
  Constant2/1 -> MinMax2/1
  Mux2/1 -> fcn1/1
  MinMax/1 -> Mux2/1
  fcn/1 -> MinMax/2
  Constant/1 -> MinMax/1
  MinMax1/1 -> Mux1/2
  c_psi1/1 -> MinMax1/1
  Constant1/1 -> MinMax1/2
  Mux1/1 -> fcn/1
  PSI_c/1 -> Mux1/1
  omega_t/1 -> c_phi1/1, c_psi1/1, Mux5/3
  T_bc/1 -> Mux5/2
  PI_c/1 -> Mux5/1
  Mux5/1 -> PSI_c/1

== system paramAB_model/Model/Engine/Turbo/Turbine/Sub W_t/f_vgt ==
  u_vgt : Inport
  Constant : Constant  Value=0
  Constant1 : Constant  Value=0
  Fcn f_vgt : Fcn  Expr=c_f2+c_f1*sqrt(u)
  Fcn1 : Fcn  Expr=1-((u-c_vgt2)/c_vgt1)^2
  MinMax : MinMax  Function=max  Inputs=2  SaturateOnIntegerOverflow=on  InputSameDT=on
  MinMax1 : MinMax  Function=max  Inputs=2  SaturateOnIntegerOverflow=on  InputSameDT=on
  f_vgt : Outport
  wires:
  MinMax1/1 -> f_vgt/1
  Fcn f_vgt/1 -> MinMax1/1
  Constant1/1 -> MinMax1/2
  MinMax/1 -> Fcn f_vgt/1
  Constant/1 -> MinMax/2
  Fcn1/1 -> MinMax/1
  u_vgt/1 -> Fcn1/1

== system paramAB_model/Model/Engine/Turbo/Turbine/eta_tm/c_m ==
  omega_t : Inport
  Constant : Constant  Value=c_mVec(2)
  MinMax : MinMax  Function=max  Inputs=2  SaturateOnIntegerOverflow=on  InputSameDT=on
  Switch PSI : Switch  Threshold=w_tlin  SaturateOnIntegerOverflow=on
  c_m linear : Fcn  Expr=c_mlin*(u-c_mVec(2))/(w_tlin-c_mVec(2))
  c_m power : Fcn  Expr=c_mVec(1)*(u-c_mVec(2))^c_mVec(3)
  c_m : Outport
  wires:
  Switch PSI/1 -> c_m/1
  c_m linear/1 -> Switch PSI/3
  c_m power/1 -> Switch PSI/1
  omega_t/1 -> MinMax/2
  Constant/1 -> MinMax/1
  MinMax/1 -> c_m linear/1, Switch PSI/2, c_m power/1
